simulink model "Model_4b_CH4_Flexible_clean"  (R2019a)
settings: Solver=FixedStepAuto  StartTime=0.0  StopTime=8760  FixedStep=1  RelTol=1e-3
libraries: simulink x6
settings Model: Creator=senja  LastModifiedBy=senja

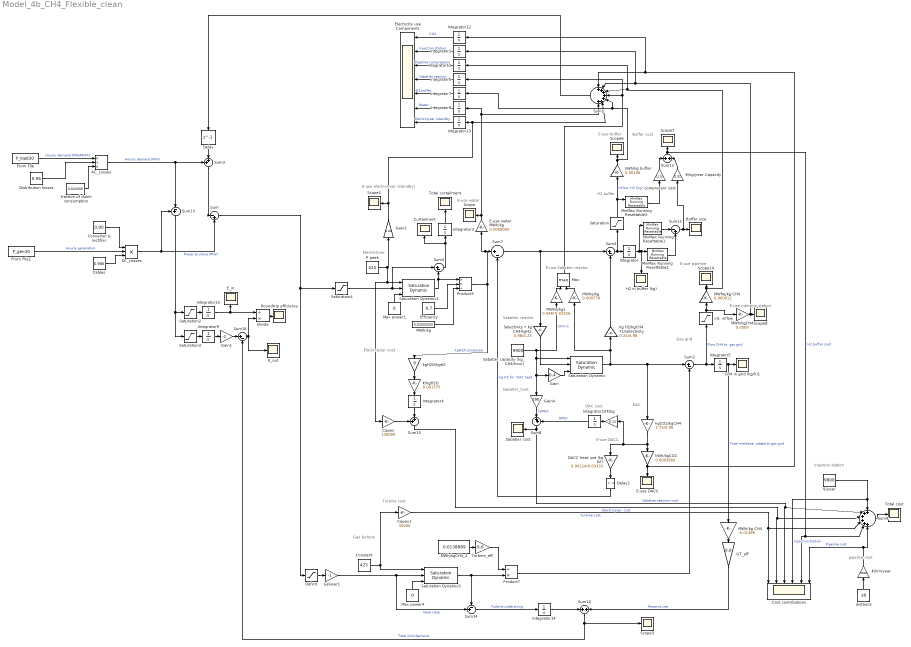
== system Model_4b_CH4_Flexible_clean ==
  note: DAC cost
  note: DAC
  note: E-use pipeline
  note: pipeline cost
  note: E-use injection station
  note: E-use buffer
  note: Buffer cost
  note: E-use Sabatier reactor
  note: E-use DACC
  note: Sabatier_Cost
  note: Injection station
  note: Gas grid
  note: Sabatier reactor
  note: E-use electrolyser (standby)
  note: E-use water
  note: Turbine cost
  note: Gas turbine
  note: Electrolyser
  note: Electrolyzer cost
  note: H2 buffer
  ">0, inflow" : Saturate  UpperLimit=inf  LowerLimit=0
  AC_Losses : Product  Inputs=*/*
  Buffer size : Scope
  CH4 in grid (kg/h)1 : Scope
  Cables : Constant  Value=0.985
  Capex : Gain  Gain=126000
  Capex1 : Gain  Gain=32000
  Constant : Constant  Value=425
  Converter & rectifier : Constant  Value=0.90
  Cost contributions : Scope  NumInputPorts=6
  Curtailment : Scope
  DACC heat use (kg h2) : Gain  Gain=0.00124/0.03333
  DC_Losses : Product  Inputs=3
  Deficit : Saturate  UpperLimit=0  LowerLimit=-inf
  Delay : Delay  DelayLength=1  InitialCondition=0
  Delay1 : Delay  DelayLength=1
  Distribution losses : Constant  Value=0.96
  Divide : Product  Inputs=/*
  E-use DACC : Scope
  E-use water MWh/kg : Gain  Gain=0.0000005
  "E_in " : Scope
  E_out : Scope
  Efficiency : Constant  Value=0.7
  Electricity use Components : Scope  NumInputPorts=7
  From File : FromFile  FileName=P_load30  SampleTime=0
  From File1 : FromFile  FileName=P_gen30  SampleTime=0
  GJ/year1 : Gain  Gain=-1
  GT_eff : Gain  Gain=0.6
  Gain : Gain  Gain=0.4
  Gain1 : Gain  Gain=-1
  Gain2 : Gain  Gain=0.02
  Gain4 : Gain  Gain=290
  H2 in buffer (kg) : Scope
  Integrator{,2..15} (15 alike) : Integrator
  MWh/kg : Constant  Value=0.03333333
  MWh/kg CH4 : Gain  Gain=-0.01389
  MWh/kgCH4 : Gain  Gain=0.0009
  MWh/kgCH4_2 : Constant  Value=0.0138889
  MWhe/kg : Gain  Gain=0.000778
  MWhe/kg CH4 : Gain  Gain=0.000012
  MWhe/kg1 : Gain  Gain=0.046*0.01556
  Max : MinMax  Function=max  Inputs=2
  Max power1 : Constant  Value=0
  Max power4 : Constant  Value=0
  MinMax Running Resettable1 : simulink/Math Operations/MinMax Running Resettable  Function=min  vinit=0.0
  MinMax Running Resettable2 : simulink/Math Operations/MinMax Running Resettable  Function=max  vinit=0.0
  MinMax Running Resettable3 : simulink/Math Operations/MinMax Running Resettable  Function=max  vinit=0.0
  P peek : Constant  Value=425
  Product3 : Product  Inputs=**/
  Product7 : Product  Inputs=/*
  Roundtrip efficiency : Scope
  Sabatier capacity (kg_CH4/hour) : Constant  Value=9900
  Sabatier cost : Scope
  Saturation : Saturate  UpperLimit=inf  LowerLimit=0
  Saturation Dynamic : simulink/Discontinuities/Saturation Dynamic  OutMin=[]  OutMax=[]  OutDataTypeStr=Inherit: Same as second input  OutDataType=fixdt(1, 16)  OutScaling=2^-10  DoSatur=off
  Saturation Dynamic1 : simulink/Discontinuities/Saturation Dynamic  OutMin=[]  OutMax=[]  OutDataTypeStr=Inherit: Same as second input  OutDataType=fixdt(1, 16)  OutScaling=2^-10  DoSatur=off
  Saturation Dynamic3 : simulink/Discontinuities/Saturation Dynamic  OutMin=[]  OutMax=[]  OutDataTypeStr=Inherit: Same as second input  OutDataType=fixdt(1, 16)  OutScaling=2^-10  DoSatur=off
  Saturation2 : Saturate  UpperLimit=inf  LowerLimit=0
  Saturation3 : Saturate  UpperLimit=0  LowerLimit=-inf
  Saturation4 : Saturate  UpperLimit=inf  LowerLimit=0
  Scope{,1,3,6..8,10} (7 alike) : Scope
  Selectivity * kg CH4/kgH2 : Gain  Gain=0.98/0.25
  Sum : Sum  Inputs=|-+
  Sum1 : Sum  Inputs=+++++++
  Sum10 : Sum  Inputs=+|+
  Sum11 : Sum  Inputs=|-+
  Sum12 : Sum  Inputs=+|+
  Sum13 : Sum  Inputs=+-|
  Sum14 : Sum  Inputs=-+|
  Sum15 : Sum  Inputs=++|
  Sum{2,4..5,7,16} (5 alike) : Sum  Inputs=|+-
  Sum3 : Sum  Inputs=++|
  Sum8 : Sum  Inputs=|++
  Sum9 : Sum  Inputs=++++++
  Total cost : Scope
  Total curtailment : Scope
  Turbine_eff. : Gain  Gain=0.6
  compressor cost : Gain  Gain=1170
  distance : Constant  Value=30
  fraction of dutch consumption : Constant  Value=0.023335
  kWh/kg buffer : Gain  Gain=0.00106
  kWh/kgCO2 : Gain  Gain=0.0003666
  kg H2/kgCH4 *1/selectivity : Gain  Gain=0.25/0.98
  kgCO2/kgCH4 : Gain  Gain=2.75/0.96
  kgH2O/kgH2 : Gain  Gain=9
  €/kg : Gain  Gain=0.11
  €/kg/year Capacity : Gain  Gain=0.31
  €/kgH2O : Gain  Gain=0.001375
  €/km/year : Gain  Gain=9000
  €/year : Constant  Value=9800
  wires:
  From File/1 -> AC_Losses/1  "Hourly demand (MW/MWh)"
  Efficiency/1 -> Product3/2
  fraction of dutch consumption/1 -> AC_Losses/3
  Distribution losses/1 -> AC_Losses/2
  Cables/1 -> DC_Losses/3
  Converter & rectifier/1 -> DC_Losses/1
  DC_Losses/1 -> Sum/2, Sum13/1  "Power to shore (MW)"
  Saturation4/1 -> Sum5/1, Saturation Dynamic1/2
  Deficit/1 -> GJ/year1/1
  AC_Losses/1 -> Sum3/1, Sum13/2  "Hourly demand (MW)"
  From File1/1 -> DC_Losses/2  "Hourly generation"
  Max power1/1 -> Saturation Dynamic1/3
  Saturation Dynamic1/1 -> Sum5/2, Product3/1
  Capex/1 -> Sum15/1
  Sum15/1 -> Sum9/3, Cost contributions/2  "Electrolyzer  cost"
  €/kgH2O/1 -> Integrator4/1
  P peek/1 -> Saturation Dynamic1/1, Capex/1, Gain2/1
  GJ/year1/1 -> Saturation Dynamic3/2, Sum14/2  "base case"
  Product3/1 -> kgH2O/kgH2/1, E-use water MWh/kg/1, Sum7/1  "kgH2/h produced"
  Sum/1 -> Saturation4/1, Deficit/1
  Sum9/1 -> Total cost/1
  Constant/1 -> Saturation Dynamic3/1, Capex1/1
  Max power4/1 -> Saturation Dynamic3/3
  Saturation Dynamic3/1 -> Sum14/1, Product7/2
  MWh/kgCH4_2/1 -> Turbine_eff./1
  Integrator3/1 -> Total curtailment/1
  kgH2O/kgH2/1 -> €/kgH2O/1
  Integrator4/1 -> Sum15/2
  MWh/kg/1 -> Product3/3
  Capex1/1 -> Cost contributions/1, Sum9/4  "Turbine cost"
  Turbine_eff./1 -> Product7/1
  Sum5/1 -> Curtailment/1, Integrator3/1
  Sum14/1 -> Integrator14/1  "Turbine undersizing"
  E-use water MWh/kg/1 -> Scope/1, Sum1/7, Integrator8/1
  Gain2/1 -> Sum1/6, Integrator13/1, Scope1/1
  Sum3/1 -> Sum/1
  Sum1/1 -> Delay/1
  Delay/1 -> Sum3/2
  Integrator2/1 -> Electricity use Components/2  "Injection station"
  Integrator6/1 -> Electricity use Components/4  "Sabatier reactor"
  Integrator7/1 -> Electricity use Components/5  "H2 buffer"
  Integrator8/1 -> Electricity use Components/6  "Water"
  Sum7/1 -> Sum4/1, Selectivity * kg CH4/kgH2/1
  Integrator/1 -> H2 in buffer (kg)/1, MinMax Running Resettable2/1, MinMax Running Resettable1/1
  Sum10/1 -> Sum16/2, Scope3/1  "Total Grid demand"
  GT_eff/1 -> Sum10/2  "Reserve use"
  Integrator5/1 -> CH4 in grid (kg/h)1/1, MWh/kg CH4/1  "Total methane  added to gas grid"
  Gain4/1 -> Sum8/1  "CAPEX"
  kgCO2/kgCH4/1 -> DACC heat use (kg h2)/1, €/kg/1, kWh/kgCO2/1
  €/kg/1 -> Integrator10/1
  Sum8/1 -> Cost contributions/3, Sum9/2, Sabatier cost/1  "Sabatier reactorr cost"
  Integrator10/1 -> Sum8/2  "OPEX"
  Max/1 -> Sum1/4, Integrator6/1
  Integrator12/1 -> Electricity use Components/1  "CO2"
  Integrator11/1 -> Electricity use Components/3  "Pipeline compressors"
  kWh/kgCO2/1 -> Integrator12/1, Sum1/1, E-use DACC/1
  MinMax Running Resettable1/1 -> Sum11/1
  MinMax Running Resettable2/1 -> Sum11/2
  Sum11/1 -> €/kg/year Capacity/1, Buffer size/1
  €/kg/year Capacity/1 -> Sum12/2
  kWh/kg buffer/1 -> Integrator7/1, Sum1/5, Scope6/1
  Saturation/1 -> kWh/kg buffer/1, MinMax Running Resettable3/1  "inflow  H2 (kg)"
  MinMax Running Resettable3/1 -> compressor cost/1
  compressor cost/1 -> Sum12/1
  Sum12/1 -> Cost contributions/5, Sum9/5, Scope7/1  "H2 buffer cost"
  Integrator13/1 -> Electricity use Components/7  "Eelctrolyser (standby"
  DACC heat use (kg h2)/1 -> Delay1/1
  Sabatier capacity (kg_CH4/hour)/1 -> MWhe/kg1/1, Saturation Dynamic/1, Gain/1, Gain4/1  "CH4 in"
  Sum2/1 -> Integrator5/1, ">0, inflow"/1  "Flow CH4 to  gas grid"
  €/year/1 -> Cost contributions/4, Sum9/1  "Injection station"
  ">0, inflow"/1 -> MWhe/kg CH4/1, MWh/kgCH4/1
  MWh/kgCH4/1 -> Integrator2/1, Sum1/2, Scope8/1
  distance/1 -> €/km/year/1
  €/km/year/1 -> Cost contributions/6, Sum9/6  "Pipeline cost"
  MWhe/kg CH4/1 -> Integrator11/1, Sum1/3, Scope10/1
  Integrator14/1 -> Sum10/1
  Selectivity * kg CH4/kgH2/1 -> Saturation Dynamic/2
  Gain/1 -> Saturation Dynamic/3
  Saturation Dynamic/1 -> kgCO2/kgCH4/1, Sum2/1, kg H2/kgCH4 *1/selectivity/1, MWhe/kg/1
  Delay1/1 -> Sum7/2  "kg H2 for  DAC heat"
  Sum4/1 -> Integrator/1, Saturation/1
  kg H2/kgCH4 *1/selectivity/1 -> Sum4/2
  MWhe/kg1/1 -> Max/1
  MWhe/kg/1 -> Max/2
  Integrator9/1 -> Gain1/1
  Sum13/1 -> Saturation2/1, Saturation3/1
  Saturation2/1 -> Integrator15/1
  Saturation3/1 -> Integrator9/1
  Integrator15/1 -> Divide/1, "E_in "/1
  Gain1/1 -> Sum16/1
  Divide/1 -> Roundtrip efficiency/1
  Sum16/1 -> Divide/2, E_out/1
  Product7/1 -> Sum2/2
  MWh/kg CH4/1 -> GT_eff/1
